simulink model "Lookuptest"  (R2022b)
settings: Solver=ode4  StartTime=0.0  StopTime=20  FixedStep=1e-4  RelTol=1e-3
values from neighbouring files (symbols this model uses):
  vartosave = struct('Current',I_sweep,'Voltage',outIV.Vfc)    [PAC_IV.m]
libraries: spsControlledCurrentSourceLib x1, spsFuelCellStackLib x1, spsVoltageMeasurementLib x1, sps_lib x1
settings Model: Creator=ZinouAb  LastModifiedBy=ZinouAb

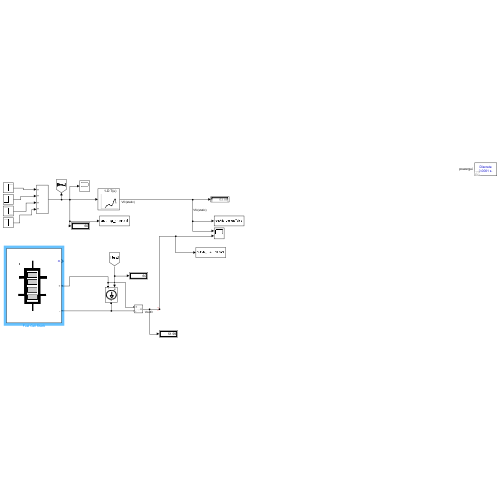
[thumbnail: Simulink's stored preview of the top-level diagram]
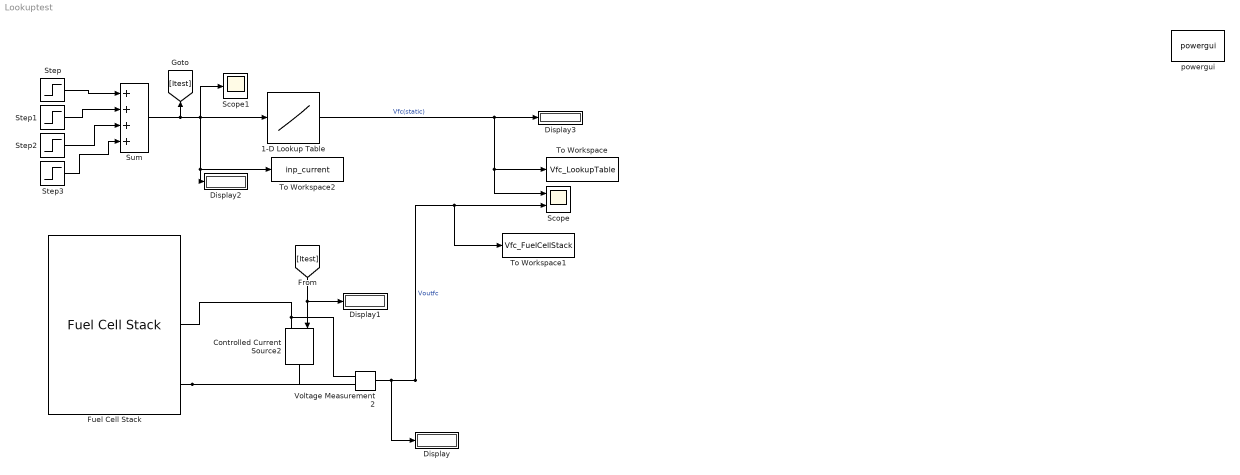
== system Lookuptest ==
  1-D Lookup Table : Lookup_n-D  NumberOfTableDimensions=1  BreakpointsForDimension1=vartosave.Current'  Table=vartosave.Voltage.Data  InterpMethod=Cubic spline  ExtrapMethod=Clip  DiagnosticForOutOfRangeInput=Error  InternalRulePriority=Speed  RndMeth=Simplest
  Controlled Current Source2 : spsControlledCurrentSourceLib/Controlled Current Source  Initialize=on  Source_Type=AC  Amplitude=0  Phase=0  Frequency=0  Measurements=None
  Display{,1..3} (4 alike) : Display
  Fuel Cell Stack : spsFuelCellStackLib/Fuel Cell Stack  PresetModel=PEMFC - 6 kW - 45 Vdc  FcType=Proton Exchange Membrane (PEM)  Detailed=Detailed  Eoc=[65,63]  NomVI=[133.3,45]  EndVI=[225,37]  Nc=65  n=55  TOp=65  AirFr=300  SuppPress=[1.5,1]  Comp=[99.95,21,1]  SignX=off  SignY=off  FlowRateH2=off  FlowRateAir=off  SystemTemp=off  SystemPH2=off  SystemPAir=off  FCDyn=on  FC_tau=1  Peak_O2=80  V_Under=10
      settings: LibrarySourceBlock=electricdrivelib/Extra Sources/Fuel Cell Stack
  Scope : Scope  NumInputPorts=2
  Scope1 : Scope
  Step : Step  After=100  SampleTime=0
  Step1 : Step  Time=7  After=30  SampleTime=0
  Step2 : Step  Time=10  After=-30  SampleTime=0
  Step3 : Step  Time=15  After=-40  SampleTime=0
  Sum : Sum  Inputs=++++
  To Workspace : ToWorkspace  VariableName=Vfc_LookupTable  SaveFormat=Timeseries  SampleTime=-1
  To Workspace1 : ToWorkspace  VariableName=Vfc_FuelCellStack  SaveFormat=Timeseries  SampleTime=-1
  To Workspace2 : ToWorkspace  VariableName=inp_current  SaveFormat=Timeseries  SampleTime=-1
  Voltage Measurement2 : spsVoltageMeasurementLib/Voltage Measurement  PhasorSimulation=off  OutputType=Complex  PSBequivalent=0
  powergui : sps_lib/powergui  Priority=1  SimulationMode=Discrete  SampleTime=1e-4  frequency=60  Iterations=50  frequencyindice=0  Pbase=100e6  ErrMax=1e-4  UnitsV=kV  UnitsW=MW  buscounter=0  FunctionMessages=off  echomessages=off  EnableUseOfTLC=off  CurrentSourceSwitches=off  DisableSnubberDevices=on  DisableRonSwitches=on  DisableVfSwitches=on  DisplayEquations=off  AutomaticDiscreteSolvers=off  SolverType=Tustin  Interpol=off  ExternalGateDelay=off  methode=off  Ts=0  x0status=blocks  SPID=on  SwTol=0  HookPort=off  NonlinearTolerance=1e-4  nMaxIteration=100  ContinueOnMaxIteration=off  RestoreLinks=warning  ResistiveCurrentMeasurement=off  Frange=[0:2:500]  Ylog=off  Xlog=on  ShowGrid=off  save=off  variable=ZData  structure=0  ZoomFFT=off  StartTime=0.0  cycles=1  DisplayStyle=1  fundamental=60  FreqAxis=off  MaxFrequency=1000  frequencyindicesteady=1  RmsSteady=1  display=off
  wires:
  Voltage Measurement2/1 -> To Workspace1/1, Scope/2, Display/1  "Voutfc"
  [Itest] -> Display1/1, Controlled Current Source2/1
  Sum/1 -> To Workspace2/1, Display2/1, Scope1/1, 1-D Lookup Table/1, [Itest]
  1-D Lookup Table/1 -> Display3/1, Scope/1, To Workspace/1  "Vfc(static)"
  Step/1 -> Sum/1
  Step1/1 -> Sum/2
  Step2/1 -> Sum/3
  Step3/1 -> Sum/4
  connections:
  Fuel Cell Stack/RConn2 -- Voltage Measurement2/LConn2 -- Controlled Current Source2/RConn1
  Fuel Cell Stack/RConn1 -- Voltage Measurement2/LConn1 -- Controlled Current Source2/LConn1
